simulink subsystem "ThrustSignals"  (R2021a)
settings: Solver=VariableStepAuto  StartTime=0.0  StopTime=10.0  RelTol=1e-3
undefined symbols (not defined in the file): t0x, t0y, t0z, t_thrust, tfx, tfy, tfz, Tmax
settings Model: Creator=Laura  LastModifiedBy=Laura

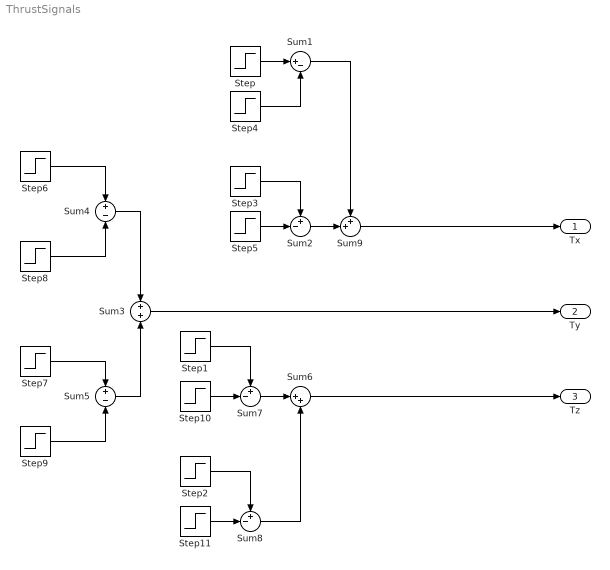
== system ThrustSignals ==
  Step : Step  Time=t0x  After=Tmax  SampleTime=0
  Step1 : Step  Time=t0z  After=Tmax  SampleTime=0
  Step10 : Step  Time=t0z + t_thrust  After=Tmax  SampleTime=0
  Step11 : Step  Time=tfz + t_thrust  After=-Tmax  SampleTime=0
  Step2 : Step  Time=tfz  After=-Tmax  SampleTime=0
  Step3 : Step  Time=tfx  After=-Tmax  SampleTime=0
  Step4 : Step  Time=t0x + t_thrust  After=Tmax  SampleTime=0
  Step5 : Step  Time=tfx + t_thrust  After=-Tmax  SampleTime=0
  Step6 : Step  Time=t0y  After=Tmax  SampleTime=0
  Step7 : Step  Time=tfy  After=-Tmax  SampleTime=0
  Step8 : Step  Time=t0y + t_thrust  After=Tmax  SampleTime=0
  Step9 : Step  Time=tfy + t_thrust  After=-Tmax  SampleTime=0
  Sum1 : Sum  Inputs=|+-
  Sum2 : Sum  Inputs=+-|
  Sum3 : Sum
  Sum4 : Sum  Inputs=+-
  Sum5 : Sum  Inputs=+-
  Sum6 : Sum  Inputs=|++
  Sum7 : Sum  Inputs=+-|
  Sum8 : Sum  Inputs=+-|
  Sum9 : Sum  Inputs=++|
  Tx : Outport
  Ty : Outport  Port=2
  Tz : Outport  Port=3
  wires:
  Step6/1 -> Sum4/1
  Sum1/1 -> Sum9/1
  Step/1 -> Sum1/1
  Sum4/1 -> Sum3/1
  Step7/1 -> Sum5/1
  Step11/1 -> Sum8/2
  Step2/1 -> Sum8/1
  Step1/1 -> Sum7/1
  Step8/1 -> Sum4/2
  Sum7/1 -> Sum6/1
  Sum5/1 -> Sum3/2
  Step3/1 -> Sum2/1
  Step5/1 -> Sum2/2
  Sum8/1 -> Sum6/2
  Step4/1 -> Sum1/2
  Step9/1 -> Sum5/2
  Step10/1 -> Sum7/2
  Sum2/1 -> Sum9/2
  Sum9/1 -> Tx/1
  Sum3/1 -> Ty/1
  Sum6/1 -> Tz/1
